simulink model "MSX60_10_by2_PandO_US"  (Simulink 7.9)
settings: Solver=FixedStepDiscrete  StartTime=0.0  StopTime=5  FixedStep=1e-3  RelTol=1e-4
model workspace (MAT data in the model file):
  Isc = 3.8
  Voc = 21.1
  Ns = 1
  Gstc = 1000
  n = 1.3
  Rs = 0.58
  D = 0.8
  Flag = 0
  Voc_array : num (value not decoded)
values from neighbouring files (symbols this model uses):
  D = { 'G=',num2str(G(1));     'Pmpp=',num2str(Pmpp);     'Vmpp=',num2str(Vmpp);     'Impp=',num2str(Impp);     'Voc=',num2str(Voc);     'Isc=',num2str(Isc); }    [MSX60DS.m]    (also in MSX60_10_by2_with_PandO.m = Dp; MSX60_10_by2_with_PandO_PS.m = Dp; MSX60_10_by2_with_PandO_US (1).m = Dp; MSX60_10_by2_with_PandO_US.m = Dp)
  n = 1.3    [MSX60DS.m]    (also in MSX60_10_RL.m; MSX60_10_by2_with_PandO.m; MSX60_10_by2_with_PandO_PS.m; MSX60_10_by2_with_PandO_US (1).m)
  Ns = 1    [MSX60DS.m]    (also in MSX60_10_RL.m; MSX60_10_by2_with_PandO.m; MSX60_10_by2_with_PandO_PS.m; MSX60_10_by2_with_PandO_US (1).m)
  Rs = 0.58    [MSX60DS.m]    (also in MSX60_10_RL.m; MSX60_10_by2_with_PandO.m; MSX60_10_by2_with_PandO_PS.m; MSX60_10_by2_with_PandO_US (1).m)
  Voc = Voc(1)    [MSX60DS.m]    (also in MSX60_10_RL.m = 21.1; MSX60_10_by2_with_PandO.m = 21.1; MSX60_10_by2_with_PandO_PS.m = 21.1; MSX60_10_by2_with_PandO_US (1).m = 21.1)
  Voc_array = Voc*N +a*Vt*N*log(G/Gstc)    [MSX60_10_by2_with_PandO.m]    (also in MSX60_10_by2_with_PandO_PS.m; MSX60_10_by2_with_PandO_US (1).m; MSX60_10_by2_with_PandO_US.m; MSX60_G1G2.m)
undefined symbols (not defined in the file or in its folder): sigbuilder_block
libraries: fl_lib x24, elec_lib x20, nesl_utility x5
settings Model: Creator=pc1  LastModifiedBy=pc1
settings SolverCC: SolverJacobianMethodControl=SparsePerturbation
settings DataIOCC: SaveState=on
settings DebuggingCC: SolverPrmCheckMsg=none

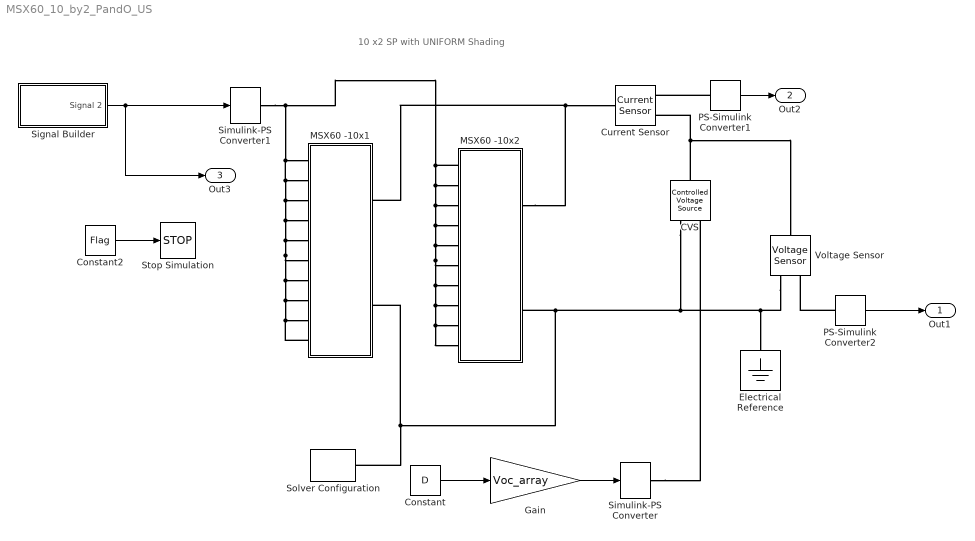
== system MSX60_10_by2_PandO_US ==
  note: 10 x2 SP with UNIFORM Shading
  CVS : fl_lib/Electrical/Electrical Sources/Controlled Voltage Source  i_Log=off  v_Log=off  LocalVarNames=|i|v  LocalVarDescs=|i|v  LocalVarLogging=[0 0]
  Constant : Constant  Value=D
  Constant2 : Constant  Value=Flag
  Current Sensor : fl_lib/Electrical/Electrical Sensors/Current Sensor  i1_Log=off  v1_Log=off  LocalVarNames=|i1|v1  LocalVarDescs=|i1|v1  LocalVarLogging=[0 0]
  Electrical Reference : fl_lib/Electrical/Electrical Elements/Electrical Reference  i_Log=off  LocalVarNames=|i  LocalVarDescs=|i  LocalVarLogging=0
  Gain : Gain  Gain=Voc_array
  MSX60 -10x1 : Subsystem
  MSX60 -10x2 : Subsystem
  PS-Simulink Converter1 : nesl_utility/PS-Simulink Converter  PhysicalDomain=network_engine_domain  LeftPortType=input  RightPortType=output  SubClassName=ps_output  Unit=1  AffineConversion=off
  PS-Simulink Converter2 : nesl_utility/PS-Simulink Converter  PhysicalDomain=network_engine_domain  LeftPortType=input  RightPortType=output  SubClassName=ps_output  Unit=1  AffineConversion=off
  Signal Builder : Subsystem  Tag=STV Subsys  LoadFcn=sigbuilder_block('load');  StartFcn=sigbuilder_block('start');  StopFcn=sigbuilder_block('stop');  ClipboardFcn=sigbuilder_block('clipboard');  mask(Sigbuilder block){}
      mask help: Simulink:masks:SigbuilderBlock_MD
      mask init:
      | if ~strcmp(get_param(bdroot(gcbh),'SimulationStatus'),'stopped') tuvar = sigbuilder_block('maskInit'); end
      settings: CopyFcn=sigbuilder_block('copy');  DeleteFcn=sigbuilder_block('delete');  ModelCloseFcn=sigbuilder_block('modelClose');  PreSaveFcn=sigbuilder_block('preSave');  PauseFcn=sigbuilder_block('pause');  ContinueFcn=sigbuilder_block('continue');  NameChangeFcn=sigbuilder_block('namechange');  OpenFcn=sigbuilder_block('open',[437.25 118.5 550.5 394.5 ]);  CloseFcn=sigbuilder_block('close');
      mask Display: plot(0, 0, 100, 100,[2, 2, 32, 32, 2], [68, 8, 8, 68, 68],[32, 2], [38, 38], [32, 19, 2],[53, 60, 44], [32, 17, 17, 2],[16, 16, 31, 31]);txt = getActiveGroup(gcbh);text(2, 100, txt,'verticalAlignment', 'top');
  Simulink-PS Converter : nesl_utility/Simulink-PS Converter  PhysicalDomain=network_engine_domain  LeftPortType=input  RightPortType=output  SubClassName=ps_input  Unit=1  AffineConversion=off  InputFilterTimeConstant=.001  UdotUserProvided=[]  SimscapeFilterOrder=1  InputFiltering=off
  Simulink-PS Converter1 : nesl_utility/Simulink-PS Converter  PhysicalDomain=network_engine_domain  LeftPortType=input  RightPortType=output  SubClassName=ps_input  Unit=1  AffineConversion=off  InputFilterTimeConstant=.001  UdotUserProvided=[]  SimscapeFilterOrder=1  InputFiltering=off
  Solver Configuration : nesl_utility/Solver Configuration  PhysicalDomain=network_engine_domain  LeftPortType=input  RightPortType=generic  SubClassName=solver  UseCustomDae=off  DoDC=on  ResidualTolerance=1e-9  UseLocalSolver=on  LocalSolverChoice=NE_TRAPEZOIDAL_ADVANCER  LocalSolverSampleTime=.001  DoFixedCost=on  MaxNonlinIter=3  MaxModeIter=2  LinearAlgebra=Sparse  Accelerate=off  Profile=off  UseLocalSampling=off  DelaysMemoryBudget=1024
  Stop Simulation : Stop
  Voltage Sensor : fl_lib/Electrical/Electrical Sensors/Voltage Sensor  i1_Log=off  v1_Log=off  LocalVarNames=|i1|v1  LocalVarDescs=|i1|v1  LocalVarLogging=[0 0]
  Out1 : Outport
  Out2 : Outport  Port=2
  Out3 : Outport  Port=3
  wires:
  PS-Simulink Converter1/1 -> Out2/1
  PS-Simulink Converter2/1 -> Out1/1
  Constant2/1 -> Stop Simulation/1
  Gain/1 -> Simulink-PS Converter/1
  Constant/1 -> Gain/1
  Signal Builder/1(Signal 2) -> Simulink-PS Converter1/1, Out3/1
  connections:
  MSX60 -10x1/LConn10 -- MSX60 -10x2/LConn1 -- MSX60 -10x2/LConn2 -- MSX60 -10x2/LConn3 -- MSX60 -10x2/LConn4 -- MSX60 -10x2/LConn5 -- MSX60 -10x2/LConn6 -- MSX60 -10x2/LConn7 -- MSX60 -10x2/LConn8 -- MSX60 -10x2/LConn10 -- MSX60 -10x2/LConn9 -- Simulink-PS Converter1/RConn1 -- MSX60 -10x1/LConn1 -- MSX60 -10x1/LConn2 -- MSX60 -10x1/LConn3 -- MSX60 -10x1/LConn4 -- MSX60 -10x1/LConn5 -- MSX60 -10x1/LConn6 -- MSX60 -10x1/LConn7 -- MSX60 -10x1/LConn8 -- MSX60 -10x1/LConn9
  Solver Configuration/RConn1 -- Voltage Sensor/RConn2 -- Electrical Reference/LConn1 -- CVS/RConn2 -- MSX60 -10x2/RConn2 -- MSX60 -10x1/RConn2
  MSX60 -10x2/RConn1 -- MSX60 -10x1/RConn1 -- Current Sensor/LConn1
  PS-Simulink Converter1/LConn1 -- Current Sensor/RConn1
  CVS/LConn1 -- Current Sensor/RConn2 -- Voltage Sensor/LConn1
  Simulink-PS Converter/RConn1 -- CVS/RConn1
  PS-Simulink Converter2/LConn1 -- Voltage Sensor/RConn1

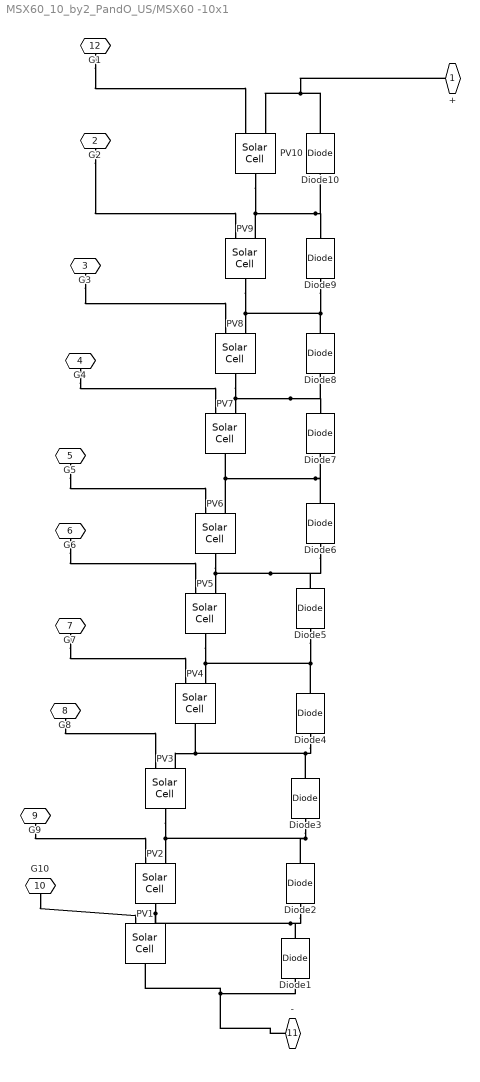
== system MSX60_10_by2_PandO_US/MSX60 -10x1 ==
  Diode{1..10} (10 alike) : fl_lib/Electrical/Electrical Elements/Diode  Vf=0.6 V  Ron=0.3 Ohm  Goff=1e-8 1/Ohm  i_Log=off  v_Log=off  LocalVarNames=|i|v  LocalVarDescs=|i|v  LocalVarLogging=[0 0]
  PV{1..10} (10 alike) : elec_lib/Sources/Solar Cell  prm=1  Isc=Isc A  Voc=Voc*Ns V  Is=1e-6 A  Is2=0 A  Iph=3.8 A  Ir0=Gstc W/m^2  ec=n*Voc*Ns  N2=0  Rs=Rs*Ns Ohm  Rp=Inf Ohm  TIPH1=0 1/K  EG=1.11 eV  TXIS1=3  TXIS2=3  TRS1=0  TRP1=0  Tmeas=25 C  TFIXED=25 C  LocalVarLogging=[]  thermal_mass=100 J/K  initial_temperature=25 C
  + : PMIOPort  Port=1  Side=Right
  G2 : PMIOPort  Port=2  Side=Left
  G3 : PMIOPort  Port=3  Side=Left
  G4 : PMIOPort  Port=4  Side=Left
  G5 : PMIOPort  Port=5  Side=Left
  G6 : PMIOPort  Port=6  Side=Left
  G7 : PMIOPort  Port=7  Side=Left
  G8 : PMIOPort  Port=8  Side=Left
  G9 : PMIOPort  Port=9  Side=Left
  G10 : PMIOPort  Port=10  Side=Left
  - : PMIOPort  Port=11  Side=Right
  G1 : PMIOPort  Port=12  Side=Left
  connections:
  Diode4/LConn1 -- PV3/LConn2 -- PV4/RConn1 -- Diode3/RConn1
  Diode5/LConn1 -- PV5/RConn1 -- PV4/LConn2 -- Diode4/RConn1
  Diode6/LConn1 -- PV6/RConn1 -- PV5/LConn2 -- Diode5/RConn1
  PV8/RConn1 -- PV7/LConn2 -- Diode7/RConn1 -- Diode8/LConn1
  Diode9/LConn1 -- PV8/LConn2 -- PV9/RConn1 -- Diode8/RConn1
  G10/RConn1 -- PV1/LConn1
  -/RConn1 -- PV1/RConn1 -- Diode1/LConn1
  G9/RConn1 -- PV2/LConn1
  Diode2/LConn1 -- PV2/RConn1 -- PV1/LConn2 -- Diode1/RConn1
  Diode3/LConn1 -- PV2/LConn2 -- PV3/RConn1 -- Diode2/RConn1
  G8/RConn1 -- PV3/LConn1
  PV6/LConn2 -- PV7/RConn1 -- Diode7/LConn1 -- Diode6/RConn1
  PV9/LConn2 -- PV10/RConn1 -- Diode9/RConn1 -- Diode10/LConn1
  Diode10/RConn1 -- PV10/LConn2 -- +/RConn1
  G7/RConn1 -- PV4/LConn1
  G6/RConn1 -- PV5/LConn1
  G5/RConn1 -- PV6/LConn1
  G4/RConn1 -- PV7/LConn1
  G3/RConn1 -- PV8/LConn1
  G2/RConn1 -- PV9/LConn1
  G1/RConn1 -- PV10/LConn1

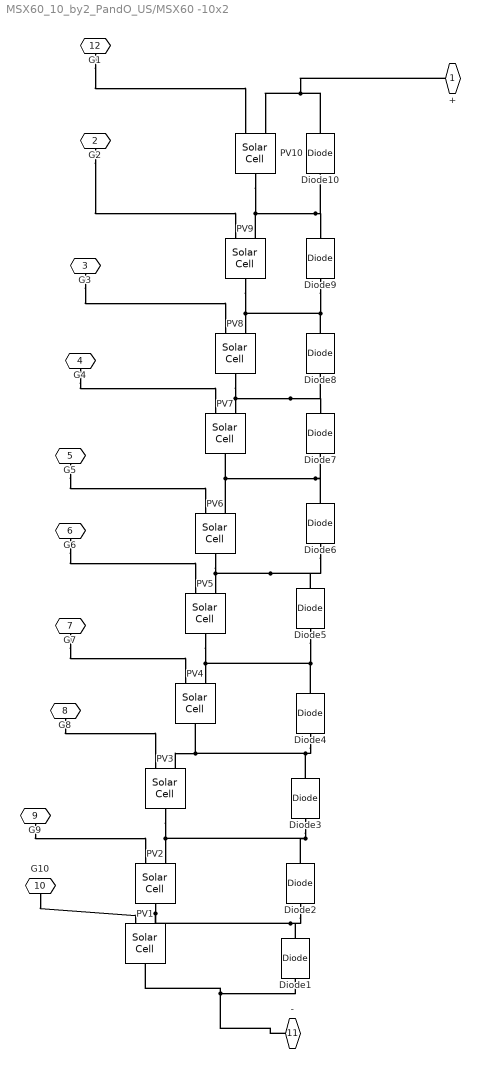
== system MSX60_10_by2_PandO_US/MSX60 -10x2 ==
  Diode{1..10} (10 alike) : fl_lib/Electrical/Electrical Elements/Diode  Vf=0.6 V  Ron=0.3 Ohm  Goff=1e-8 1/Ohm  i_Log=off  v_Log=off  LocalVarNames=|i|v  LocalVarDescs=|i|v  LocalVarLogging=[0 0]
  PV{1..10} (10 alike) : elec_lib/Sources/Solar Cell  prm=1  Isc=Isc A  Voc=Voc*Ns V  Is=1e-6 A  Is2=0 A  Iph=3.8 A  Ir0=Gstc W/m^2  ec=n*Voc*Ns  N2=0  Rs=Rs*Ns Ohm  Rp=Inf Ohm  TIPH1=0 1/K  EG=1.11 eV  TXIS1=3  TXIS2=3  TRS1=0  TRP1=0  Tmeas=25 C  TFIXED=25 C  LocalVarLogging=[]  thermal_mass=100 J/K  initial_temperature=25 C
  + : PMIOPort  Port=1  Side=Right
  G2 : PMIOPort  Port=2  Side=Left
  G3 : PMIOPort  Port=3  Side=Left
  G4 : PMIOPort  Port=4  Side=Left
  G5 : PMIOPort  Port=5  Side=Left
  G6 : PMIOPort  Port=6  Side=Left
  G7 : PMIOPort  Port=7  Side=Left
  G8 : PMIOPort  Port=8  Side=Left
  G9 : PMIOPort  Port=9  Side=Left
  G10 : PMIOPort  Port=10  Side=Left
  - : PMIOPort  Port=11  Side=Right
  G1 : PMIOPort  Port=12  Side=Left
  connections:
  Diode4/LConn1 -- PV3/LConn2 -- PV4/RConn1 -- Diode3/RConn1
  Diode5/LConn1 -- PV5/RConn1 -- PV4/LConn2 -- Diode4/RConn1
  Diode6/LConn1 -- PV6/RConn1 -- PV5/LConn2 -- Diode5/RConn1
  PV8/RConn1 -- PV7/LConn2 -- Diode7/RConn1 -- Diode8/LConn1
  Diode9/LConn1 -- PV8/LConn2 -- PV9/RConn1 -- Diode8/RConn1
  G10/RConn1 -- PV1/LConn1
  -/RConn1 -- PV1/RConn1 -- Diode1/LConn1
  G9/RConn1 -- PV2/LConn1
  Diode2/LConn1 -- PV2/RConn1 -- PV1/LConn2 -- Diode1/RConn1
  Diode3/LConn1 -- PV2/LConn2 -- PV3/RConn1 -- Diode2/RConn1
  G8/RConn1 -- PV3/LConn1
  PV6/LConn2 -- PV7/RConn1 -- Diode7/LConn1 -- Diode6/RConn1
  PV9/LConn2 -- PV10/RConn1 -- Diode9/RConn1 -- Diode10/LConn1
  Diode10/RConn1 -- PV10/LConn2 -- +/RConn1
  G7/RConn1 -- PV4/LConn1
  G6/RConn1 -- PV5/LConn1
  G5/RConn1 -- PV6/LConn1
  G4/RConn1 -- PV7/LConn1
  G3/RConn1 -- PV8/LConn1
  G2/RConn1 -- PV9/LConn1
  G1/RConn1 -- PV10/LConn1

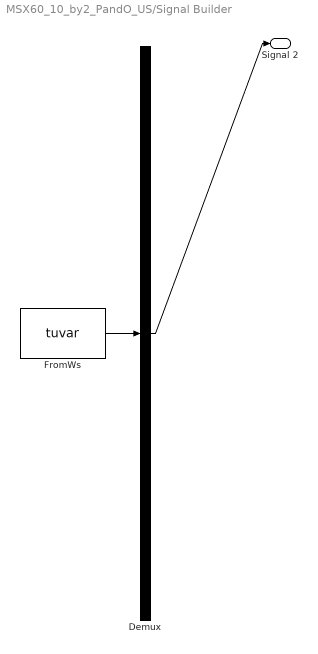
== system MSX60_10_by2_PandO_US/Signal Builder ==
  Demux : Demux  Tag=STV Demux  Outputs=1
  FromWs : FromWorkspace  Tag=STV FromWs  VariableName=tuvar  SampleTime=0  SigBuilderData=DataTag1  VnvData=DataTag2
      SigBuilderData=|
      | common.afterFinalStr = 'Extrapolate'
      | common.sampleTime = 0
      | dataSet.timeRange = [0 10]
      | dataSet.name = 'Group 1'
      | sbobj.Groups.Name = 'Group 1'
      | sbobj.Groups.Signals.Name = 'Signal 2'
      | sbobj.Groups.Signals.XData = [0 0.9999 0.9999 1.01 2 2.01 3 3.01 10]
      | sbobj.Groups.Signals.YData = [500 500 505 1000 1000 700 700 400 400]
  Signal 2 : Outport  Tag=STV Outport
  wires:
  FromWs/1 -> Demux/1
  Demux/1 -> Signal 2/1
